simulink model "SpringDamp"  (R2023a)
settings: Solver=VariableStepAuto  StartTime=0.0  StopTime=10.0  RelTol=1e-3
values from neighbouring files (symbols this model uses):
  Kd = 0.01    [SpringDamp_c.m]
  Ks = 0.02    [SpringDamp_c.m]
  m = 65    [SpringDamp_c.m]
settings Model: Creator=paragmraw  LastModifiedBy=paragmraw

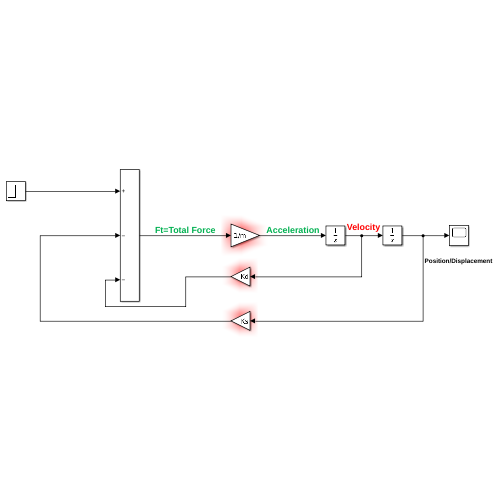
[thumbnail: Simulink's stored preview of the top-level diagram]
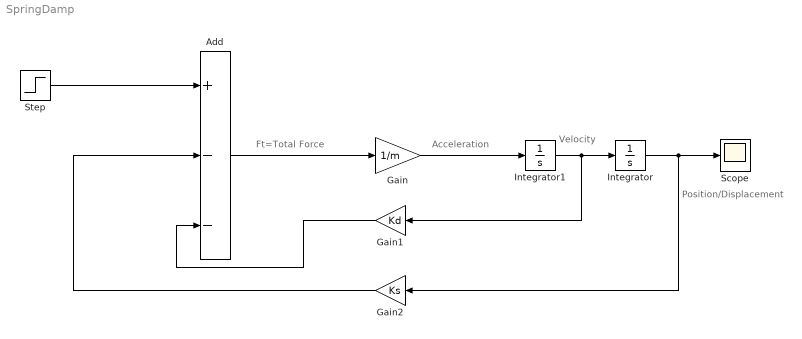
== system SpringDamp ==
  note: Ft=Total Force
  note: Acceleration
  note: Velocity
  note: Position/Displacement
  Add : Sum  Inputs=+--
  Gain : Gain  Gain=1/m
  Gain1 : Gain  Gain=Kd
  Gain2 : Gain  Gain=Ks
  Integrator : Integrator
  Integrator1 : Integrator
  Scope : Scope
  Step : Step  SampleTime=0
  wires:
  Integrator/1 -> Gain2/1, Scope/1
  Integrator1/1 -> Gain1/1, Integrator/1
  Gain/1 -> Integrator1/1
  Add/1 -> Gain/1
  Gain2/1 -> Add/2
  Gain1/1 -> Add/3
  Step/1 -> Add/1
